simulink model "Fig26"  (Simulink 8.3)
settings: Solver=ode3  StartTime=0.0  StopTime=5.24288  FixedStep=2e-5  RelTol=1e-5
libraries: commrandsrc2 x1
settings Model: Creator=Dennis Silage  LastModifiedBy=Silage
settings OptimizationCC: ExpressionDepthLimit=2147483647  InitFltsAndDblsToZero=on
settings DebuggingCC: SolverPrmCheckMsg=none  FcnCallInpInsideContextMsg=UseLocalSettings

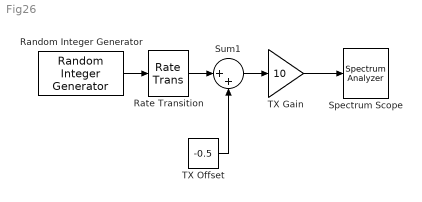
== system Fig26 ==
  Random Integer Generator : commrandsrc2/Random Integer Generator  mul=2  seed=randseed  Ts=1e-3  frameBased=off  sampPerFrame=50  orient=on  outDataType=double
  Rate Transition : RateTransition  OutPortSampleTime=2e-5
  Spectrum Scope : SpectrumAnalyzer  ScopeSpecification=DataTag0
  Sum1 : Sum  Inputs=|++
  TX Gain : Gain  Gain=10
  TX Offset : Constant  Value=-0.5
  wires:
  Random Integer Generator/1 -> Rate Transition/1
  Rate Transition/1 -> Sum1/1
  Sum1/1 -> TX Gain/1
  TX Offset/1 -> Sum1/2
  TX Gain/1 -> Spectrum Scope/1
